simulink model "ECE675_HW3_Problem3_sim"  (R2025b)
settings: Solver=VariableStepAuto  StartTime=0.0  StopTime=10.0  RelTol=1e-3
values from neighbouring files (symbols this model uses):
  x0 = x_next    [ECE675_HW3.m]    (also in ECE675_HW3_v2.m = [pi/2; 0]; ECE675_HW3_v3.m = [pi/2; 0])
undefined symbols (not defined in the file or in its folder): Ad_lin, Bd_lin, Dd_lin, K_dlqr, ts
settings Model: Creator=iwant  LastModifiedBy=iwant

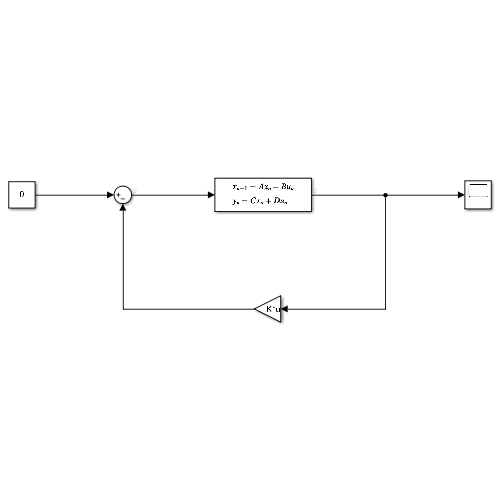
[thumbnail: Simulink's stored preview of the top-level diagram]
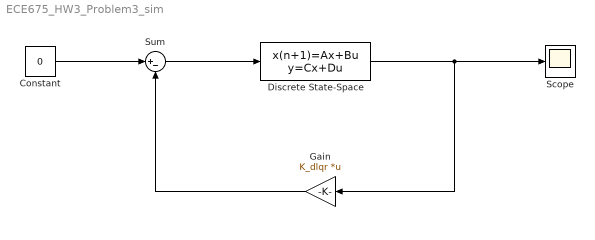
== system ECE675_HW3_Problem3_sim ==
  Constant : Constant  Value=0
  Discrete State-Space : DiscreteStateSpace  A=Ad_lin  B=Bd_lin  C=eye(2,2)  D=Dd_lin  InitialCondition=x0  SampleTime=ts
  Gain : Gain  Gain=K_dlqr  Multiplication=Matrix(K*u)
  Scope : Scope
      settings: ActiveDisplayYMinimum=-0.97205175262668742  ActiveDisplayYMaximum=0.93271015213521746
  Sum : Sum  Inputs=|+-
  wires:
  Discrete State-Space/1 -> Scope/1, Gain/1
  Gain/1 -> Sum/2
  Constant/1 -> Sum/1
  Sum/1 -> Discrete State-Space/1
